simulink model "RefModel_Navfilter"  (R2020b)
settings: Solver=ode1  StartTime=0.0  StopTime=inf  FixedStep=Ts_Navi.Ts_Base  RelTol=1e-3
values from neighbouring files (symbols this model uses):
  NAVI_PARAM_V10 = INIT_Navi_V10(NaviSimParam.Ts_Base)    [SetAlgoParam_Navi.m]
  NAVI_PARAM_V1000 = INIT_Navi_V1000(NaviSimParam.Ts_Base)    [SetAlgoParam_Navi.m]
undefined symbols (not defined in the file or in its folder): ENUM_SensorHealthStatus, NAVI_PARAM_BASE
libraries: aerolibobsolete x1
(part 2 of 2)

== stateflow chart RefModel_Navfilter/Filter_Stateflow ==
  state NaviPlatform
    en:
    initOutputData();
    initMember();
    en,du:
    % 获取输入数据
    getTaskData();
    getSensorData();
    getIntegrityData();
    % 公共状态更新
    updateMember();
    upDataOutputData();
    state LogData [parallel]
      en:
      settings: executionOrder=1
      state Work
        en,du:
        du_func_commonInfo;
        du_func_updateLog;
      (default) -> NaviPlatform.LogData.Work
    state Normal [parallel]
      en,du:
      settings: executionOrder=3
      state InitialWait0
        ex:
        mThis_RTInfo = ENUM_RTInfo_Navi.InitialWait_1_Complete; % 更新RT信息
        updateLogDataBuffer(ENUM_NaviLogBlockName.NAVILOG_Init,mThis_RTInfo,'write',double([mSensor_ublox1_pdop, mSensor_ublox1_numSv, mSensor_ublox1_pacc])); % 更新log缓存
      state InitialWait1
        ex:
        mThis_RTInfo = ENUM_RTInfo_Navi.InitialWait_2_Complete; % 更新RT信息
        updateLogDataBuffer(ENUM_NaviLogBlockName.NAVILOG_Init,mThis_RTInfo,'write',double([mSensor_ublox1_pdop, mSensor_ublox1_numSv, mSensor_ublox1_pacc])); % 更新log缓存
      state InitialAlignment
        en:
        du:
        % 执行初始化，完成滤波器初始状态的确定
        NaviFilterOut.Status.initialAlignmentComplete = coarseAlignment();
        NaviFilterOut.magDec_deg = magDec_deg;
        NaviFilterOut.Status.initNotComplete = 1;
        ex:
        NaviFilterOut.Status.initNotComplete = 0;
        mThis_RTInfo = ENUM_RTInfo_Navi.InitialWait_2_Complete; % 更新RT信息
        updateLogDataBuffer(ENUM_NaviLogBlockName.NAVILOG_Init,mThis_RTInfo,'write',[NaviFilterOut.InitValue.lla0(1:2),NaviFilterOut.InitValue.eulerd0]); % 更新log缓存
      state RunKalmanFilter
        en:
        du:
        du_func_KalmanFilter(NAVIParam.modeKF1); % marg mvo
      (default) -> InitialWait0
      InitialWait0 -> InitialWait1 : [isUbloxGoodForAWhile()]
      InitialWait1 -> InitialAlignment : [after(10,sec) && isUbloxGood()]
      InitialAlignment -> RunKalmanFilter : [isInitComplete()]
    state Radar [parallel]
      % 用于降落阶段雷达高度融合
      settings: executionOrder=2
      state StandBy
        en:
        resetRadarFuser = true;
      state Work
        en:
        height0Ublox1 = double(IN_Sensor.ublox1.height) - double(IN_Sensor.radar1.Range);
        height0Um482 = double(IN_Sensor.um482.height) - double(IN_Sensor.radar1.Range);
        height0Baro1 = double(IN_Sensor.baro1.alt_baro) - double(IN_Sensor.radar1.Range);
        du:
        du_func;
      (default) -> StandBy
      StandBy -> NaviPlatform.Radar.Work : [isRadarReady && after(0.1,sec)]
      NaviPlatform.Radar.Work -> StandBy : [~isRadarReady && after(2,sec)]
  data: blockName function_input; message function_input; operation function_input; varargin function_input; accel function_output; gyro function_output; imuUpdateFlag function_output; flag function_output; flag function_output; vel function_input; flag function_output; flag function_output; heading function_input; heading_ecompass function_input; flag function_output; isSuccess function_output; mode function_input; flag function_output; x_out function_output; Vd function_input; height function_input; Ts_in function_input; P_out function_output; dz_out function_output; Pz_out function_output; reset function_input; reject_threshold function_input; Q function_input; R function_input; mode function_input; mag function_output; magUpdateFlag function_output; isBagMag function_output; tas function_output; airspeedUpdateFlag function_output; alt function_output; baroUpdateFlag function_output; range function_output; radarUpdateFlag function_output; out function_output; Ts input; clock_sec input; magDec_deg input; IN_Sensor input Bus: BUS_SENSOR; IN_SignalIntegrity input Bus: BUS_NAVI_SensorSignalIntegrity; IN_Task input size=1; mThis_bestpos local Enum: ENUM_BESTPOS; isBadAttitude local; resetRadarFuser local; RadarFilterOut output Bus: BUS_NAVI_RadarFilter size=1; MVOParam data_store_memory; height0Baro1 local; height0Ublox1 local; height0Um482 local; NaviFilterOut output Bus: BUS_NAVI_FilterOut size=1; MARGParam data_store_memory; NAVIParam data_store_memory; isDebugInfoToShow data_store_memory; mThis_RTInfo local Enum: ENUM_RTInfo_Navi =ENUM_RTInfo_Navi(0); logDataBuffer output Bus: BUS_NAVI_SingleLog size=32; logDataOut output Bus: BUS_NAVI_SingleLog size=1; mSensor_radar1_range local; mSensor_baro1_alt local; mSensor_airspeed1_ias local; mSensor_um482_bestpos local; mSensor_IMU1_acc local; mSensor_IMU1_gyro local; mSensor_IMU2_acc local; mSensor_IMU3_acc local; mSensor_IMU2_gyro local; mSensor_IMU3_gyro local; mSensor_mag1_mag local; mSensor_mag2_mag local; mSensor_ublox1_lla local; mSensor_ublox1_ll local; mSensor_ublox1_lat local; mSensor_ublox1_lon local; mSensor_ublox1_gpsvel local; mSensor_ublox1_vd local; mSensor_ublox1_alt local; mSensor_ublox1_pdop local; mSensor_ublox1_pacc local; mSensor_ublox1_sacc local; mSensor_ublox1_numSv local; mSensor_ublox1_groundSpeed local; mSensor_airspeed2_ias local; mSensor_airspeed3_ias local; mSensor_um482_lat local; mSensor_um482_lon local; mSensor_um482_alt local; mSensor_um482_lla local; mSensor_um482_ll local; mSensor_um482_gpsvel local; mSensor_um482_groundSpeed local; mSensor_um482_vd local; mSensor_um482_pdop local; mSensor_um482_pacc local; mSensor_um482_numSv local; mIntegrity_select_IMU local; mIntegrity_statusSystemHealth local; mIntegrity_status_radar1 local; mIntegrity_status_ublox1 local; mIntegrity_status_um482 local; mIntegrity_status_airspeed1 local; mIntegrity_select_mag local; mIntegrity_select_airspeed local; mIntegrity_select_baro local; mIntegrity_select_radar local; mIntegrity_select_camera local; mIntegrity_status_mag1 local; mIntegrity_status_mag2 local; mIntegrity_status_IMU1 local; mIntegrity_status_IMU2 local; mIntegrity_status_IMU3 local; mIntegrity_status_airspeed2 local; mIntegrity_update_IMU1 local; mIntegrity_update_IMU2 local; mIntegrity_update_IMU3 local; mIntegrity_update_mag1 local; mIntegrity_update_mag2 local; mIntegrity_update_ublox1 local; mIntegrity_update_um482 local; mIntegrity_update_baro1 local; data local; mIntegrity_update_radar1 local; mIntegrity_update_radar2 local; mIntegrity_update_radar3 local; mIntegrity_update_airspeed1 local; mIntegrity_update_airspeed2 local; mIntegrity_update_airspeed3 local; mIntegrity_status_baro1 local; mTask_taskMode local
  function initOutputData:
    | function initOutputData
    | % 输出结构体进行赋值，避免报"调用前没有赋值"的错误，每个结构体赋值1个成员即可
    | NaviFilterOut.Status.initNotComplete = int8(1);
    | logDataOut(1).time_sec = 0;
    | logDataBuffer(1).time_sec = 0;
  function initMember:
    | function initMember()
    | % 初始化成员变量
  function upDataOutputData:
    | function upDataOutputData
    | % 
    | NaviFilterOut.magDec_deg = magDec_deg;
    | NaviFilterOut.hitGroundByAccZ = isHitGround(mSensor_IMU1_acc,Ts);
    | 
    | %% 子函数
    | function flag = isHitGround(acc, Ts)
    | persistent duration
    | if isempty(duration)
    |     duration = 0;
    | end
    | hitSuccess = acc(3)>14;
    | flag = true;
    | if not( hitSuccess ) 
    |     duration = duration + Ts;
    |     if duration > 0.5 % 没有出现大az一段时间后,false
    |         flag = false;
    |     end 
    | else % 出现大az，true
    |     flag = true;
    |     duration = 0;
    | end
  function updateMember:
    | function updateMember()
    | %% 每时刻均需计算的成员在此计算，大部分成员在子级模块中更新
    | %% 更新成员变量
    | mThis_bestpos = enumBESTPOS();
  function getIntegrityData:
    | function getIntegrityData()
    | % 输入结构体
    | %% 直接量
    | % 通道选择
    | mIntegrity_select_IMU = IN_SignalIntegrity.SensorSelect.IMU;
    | mIntegrity_select_mag = IN_SignalIntegrity.SensorSelect.Mag;
    | mIntegrity_select_airspeed = IN_SignalIntegrity.SensorSelect.Airspeed;
    | mIntegrity_select_baro = IN_SignalIntegrity.SensorSelect.Baro;
    | mIntegrity_select_radar = IN_SignalIntegrity.SensorSelect.Radar;
    | mIntegrity_select_camera = IN_SignalIntegrity.SensorSelect.Camera;
    | % 健康状态
    | mIntegrity_statusSystemHealth = IN_SignalIntegrity.SystemHealthStatus;
    | 
    | mIntegrity_status_IMU1 = IN_SignalIntegrity.SensorStatus.IMU1;
    | mIntegrity_status_IMU2 = IN_SignalIntegrity.SensorStatus.IMU2;
    | mIntegrity_status_IMU3 = IN_SignalIntegrity.SensorStatus.IMU3;
    | mIntegrity_status_mag1 = IN_SignalIntegrity.SensorStatus.mag1;
    | mIntegrity_status_mag2 = IN_SignalIntegrity.SensorStatus.mag2;
    | mIntegrity_status_radar1 = IN_SignalIntegrity.SensorStatus.radar1;
    | mIntegrity_status_baro1 = IN_SignalIntegrity.SensorStatus.baro1;
    | mIntegrity_status_ublox1 = IN_SignalIntegrity.SensorStatus.ublox1;
    | mIntegrity_status_um482 = IN_SignalIntegrity.SensorStatus.um482;
    | mIntegrity_status_airspeed1 = IN_SignalIntegrity.SensorStatus.airspeed1;
    | % 更新标志
    | mIntegrity_update_IMU1 = IN_SignalIntegrity.SensorUpdateFlag.IMU1;
    | mIntegrity_update_IMU2 = IN_SignalIntegrity.SensorUpdateFlag.IMU2;
    | mIntegrity_update_IMU3 = IN_SignalIntegrity.SensorUpdateFlag.IMU3;
    | mIntegrity_update_mag1 = IN_SignalIntegrity.SensorUpdateFlag.mag1;
    | mIntegrity_update_mag2 = IN_SignalIntegrity.SensorUpdateFlag.mag2;
    | mIntegrity_update_ublox1 = IN_SignalIntegrity.SensorUpdateFlag.ublox1;
    | mIntegrity_update_um482 = IN_SignalIntegrity.SensorUpdateFlag.um482;
    | mIntegrity_update_baro1 = IN_SignalIntegrity.SensorUpdateFlag.baro1;
    | mIntegrity_update_radar1 = IN_SignalIntegrity.SensorUpdateFlag.radar1;
    | mIntegrity_update_radar2 = IN_SignalIntegrity.SensorUpdateFlag.radar2;
    | mIntegrity_update_radar3 = IN_SignalIntegrity.SensorUpdateFlag.radar3;
    | mIntegrity_update_airspeed1 = IN_SignalIntegrity.SensorUpdateFlag.airspeed1;
    | mIntegrity_update_airspeed2 = IN_SignalIntegrity.SensorUpdateFlag.airspeed2;
    | mIntegrity_update_airspeed3 = IN_SignalIntegrity.SensorUpdateFlag.airspeed3;
    | %% 间接量
  function getSensorData:
    | function getSensorData
    | %% 输入结构体
    | %% 直接量
    | % IMU
    | mSensor_IMU1_az = IN_Sensor.IMU1.accel_z;
    | mSensor_IMU1_acc = double([IN_Sensor.IMU1.accel_x,IN_Sensor.IMU1.accel_y,IN_Sensor.IMU1.accel_z]);
    | mSensor_IMU2_acc = double([IN_Sensor.IMU2.accel_x,IN_Sensor.IMU2.accel_y,IN_Sensor.IMU2.accel_z]);
    | mSensor_IMU3_acc = double([IN_Sensor.IMU3.accel_x,IN_Sensor.IMU3.accel_y,IN_Sensor.IMU3.accel_z]);
    | 
    | mSensor_IMU1_gyro = double([IN_Sensor.IMU1.gyro_x,IN_Sensor.IMU1.gyro_y,IN_Sensor.IMU1.gyro_z]);
    | mSensor_IMU2_gyro = double([IN_Sensor.IMU2.gyro_x,IN_Sensor.IMU2.gyro_y,IN_Sensor.IMU2.gyro_z]);
    | mSensor_IMU3_gyro = double([IN_Sensor.IMU3.gyro_x,IN_Sensor.IMU3.gyro_y,IN_Sensor.IMU3.gyro_z]);
    | % 磁力计
    | mSensor_mag1_mag = double([IN_Sensor.mag1.mag_x, IN_Sensor.mag1.mag_y, IN_Sensor.mag1.mag_z]);
    | mSensor_mag2_mag = double([IN_Sensor.mag2.mag_x, IN_Sensor.mag2.mag_y, IN_Sensor.mag2.mag_z]);
    | % 雷达高度计
    | mSensor_radar1_range = double(IN_Sensor.radar1.Range);
    | % 气压高度计
    | mSensor_baro1_alt = double(IN_Sensor.baro1.alt_baro);
    | % 空速计
    | mSensor_airspeed1_ias = double(IN_Sensor.airspeed1.airspeed_indicate);
    | mSensor_airspeed2_ias = double(IN_Sensor.airspeed2.airspeed_indicate);
    | mSensor_airspeed3_ias = double(IN_Sensor.airspeed3.airspeed_indicate);
    | % um482
    | mSensor_um482_bestpos = IN_Sensor.um482.BESTPOS;
    | % ublox
    | gpsStruct = IN_Sensor.ublox1;
    | mSensor_ublox1_lat = double(gpsStruct.Lat);
    | mSensor_ublox1_lon = double(gpsStruct.Lon);
    | mSensor_ublox1_alt = double(gpsStruct.height);
    | mSensor_ublox1_lla = [mSensor_ublox1_lat, mSensor_ublox1_lon, mSensor_ublox1_alt];
    | mSensor_ublox1_ll = [mSensor_ublox1_lat, mSensor_ublox1_lon];
    | mSensor_ublox1_gpsvel = double([gpsStruct.velN, gpsStruct.velE, gpsStruct.velD]);
    | mSensor_ublox1_groundSpeed = norm(mSensor_ublox1_gpsvel);
    | mSensor_ublox1_vd = double(gpsStruct.velD);
    | mSensor_ublox1_pdop = gpsStruct.pDop;
    | mSensor_ublox1_pacc = double([gpsStruct.hAcc,gpsStruct.hAcc,gpsStruct.vAcc]);
    | mSensor_ublox1_sacc = double(gpsStruct.sAcc);
    | mSensor_ublox1_numSv = gpsStruct.numSv;
    | % um482
    | gpsStruct = IN_Sensor.um482;
    | mSensor_um482_lat = double(gpsStruct.Lat);
    | mSensor_um482_lon = double(gpsStruct.Lon);
    | mSensor_um482_alt = double(gpsStruct.height);
    | mSensor_um482_lla = [mSensor_um482_lat, mSensor_um482_lon, mSensor_um482_alt];
    | mSensor_um482_ll = [mSensor_um482_lat, mSensor_um482_lon];
    | mSensor_um482_gpsvel = double([gpsStruct.velN, gpsStruct.velE, gpsStruct.velD]);
    | mSensor_um482_groundSpeed = norm(mSensor_um482_gpsvel);
    | mSensor_um482_vd = double(gpsStruct.velD);
    | mSensor_um482_pdop = double(gpsStruct.pDop);
    | mSensor_um482_pacc = double([gpsStruct.delta_lat,gpsStruct.delta_lon,gpsStruct.delta_height]);
    | mSensor_um482_numSv = gpsStruct.numSv;
    | mSensor_um482_bestpos = gpsStruct.BESTPOS;
    | %% 间接量
  function getTaskData:
    | function getTaskData()
    | %% 输入结构体
    | %% 直接量
    | mTask_taskMode = IN_Task.flightTaskMode;
    | %% 间接量
  function updateLogDataBuffer(blockName,message,operation,varargin):
    | function updateLogDataBuffer(blockName,message,operation,varargin)
    | persistent pIdx pBufferIdx preTime
    | if isempty(pIdx)
    |     pIdx = 0;
    |     pBufferIdx = 0;
    |     preTime = clock_sec;
    | end
    | %%
    | if nargin == 4
    |     var_input = reshape(varargin{1},5,1);
    | else
    |     var_input = zeros(5,1);
    | end
    | bufferIdx = pBufferIdx;
    | idx = pIdx;
    | thisTime = clock_sec;
    | switch operation
    |     case 'write'
    |         thisTime = clock_sec;
    |         if preTime ~= thisTime
    |             idx = 0; % 同一时间刻度下, 不同信息的先后顺序
    |         end
    |         if bufferIdx < length(logDataBuffer)
    |             bufferIdx = bufferIdx + 1;
    |             idx = idx + 1;
    |             temp = formatLogStruct(blockName,message,var_input);
    |             tempData.time_sec = clock_sec;
    |             tempData.idx = idx;
    |             tempData.blockName = blockName;
    |             tempData.message = message;
    |             tempData.var1 = temp.var1;
    |             logDataBuffer(bufferIdx) = tempData;            
    |         end
    |     case 'read'
    |         for i_out = 1:1 %AlgoParams.logDataOutSize
    |             %             logDataOut(i_out) = resetLogStruct; % 置零
    |             logDataOut(i_out).time_sec = 0;
    |             logDataOut(i_out).idx = 0;
    |             logDataOut(i_out).blockName = ENUM_NaviLogBlockName(0);
    |             logDataOut(i_out).message = ENUM_RTInfo_Navi(0);
    |             logDataOut(i_out).var1 = zeros(5,1);
    |             if bufferIdx > 0
    |                 % 读取当前数据
    |                 logDataOut(i_out) = logDataBuffer(bufferIdx);
    |                 %                 logDataBuffer(bufferIdx) = resetLogStruct;
    | %                 fprintf('read time \t idx \t block \t message \t var1\n%.3f \t %.0f \t %d \t %d \t %.3f\n',...
    | %                     logDataBuffer(bufferIdx).time_sec,...
    | %                     logDataBuffer(bufferIdx).idx,...
    | %                     int16(logDataBuffer(bufferIdx).blockName),...
    | %                     int16(logDataBuffer(bufferIdx).message),...
    | %                     logDataBuffer(bufferIdx).var1(1));
    |                 % 将当前位置数据置零
    |                 logDataBuffer(bufferIdx).time_sec = 0;
    |                 logDataBuffer(bufferIdx).idx = 0;
    |                 logDataBuffer(bufferIdx).blockName = ENUM_NaviLogBlockName(0);
    |                 logDataBuffer(bufferIdx).message = ENUM_RTInfo_Navi(0);
    |                 logDataBuffer(bufferIdx).var1 = zeros(5,1);
    |                 bufferIdx = bufferIdx - 1;
    |             end
    |         end
    | end
    | % fprintf("logbuffer  %d / %d\n", int16(bufferIdx), int16(length(logDataBuffer)));
    | preTime = thisTime;
    | pBufferIdx = bufferIdx;
    | pIdx = idx;
    | %% 子函数
    | function log = formatLogStruct(blockName,message,var_input)
    | log.message = message;
    | log.var1 = zeros(5,1);
    | % switch blockName
    | %     case ENUM_TaskLogBlockName.TASKLOG_FlightMode
    | %         log.var1(1) = ComFlightOut.curLLA(1);
    | %         log.var1(2) = ComFlightOut.curLLA(2);
    | %         log.var1(3) = ComFlightOut.curLLA(3);
    | %         log.var1(4) = norm(ComFlightOut.curAirSpeed);
    | %         log.var1(5) = PathModeOut.uavMode;
    | % end
    | % log.var1(5) = double(IN_Mav.mavlink_msg_mission_current(1).remaining)/100;
    | if sum(var_input) ~= 0
    |     log.var1 = var_input; % 输入的优先级高
    | end
  function [accel,gyro,imuUpdateFlag] = getScreeningIMU:
    | function [accel,gyro,imuUpdateFlag] = getScreeningIMU()
    | if mIntegrity_select_IMU == 1
    |     imuUpdateFlag = mIntegrity_update_IMU1;
    |     accel = mSensor_IMU1_acc;
    |     gyro = mSensor_IMU1_gyro;
    | elseif mIntegrity_select_IMU == 2
    |     imuUpdateFlag = mIntegrity_update_IMU2;
    |     accel = mSensor_IMU2_acc;
    |     gyro = mSensor_IMU2_gyro;
    | elseif mIntegrity_select_IMU == 3
    |     imuUpdateFlag = mIntegrity_update_IMU3;
    |     accel = mSensor_IMU3_acc;
    |     gyro = mSensor_IMU3_gyro;
    | elseif mIntegrity_select_IMU == 0
    |     imuUpdateFlag = mIntegrity_update_IMU1 || mIntegrity_update_IMU2 || mIntegrity_update_IMU3;
    |     accel = (mSensor_IMU1_acc+mSensor_IMU2_acc+mSensor_IMU3_acc)/3;
    |     gyro = (mSensor_IMU1_gyro+mSensor_IMU2_gyro+mSensor_IMU3_gyro)/3;
    | else
    |     imuUpdateFlag = true;
    |     accel = [0,0,0];
    |     gyro = [0,0,0];
    |     error('IMU config error')
    | end
  function du_func_commonInfo:
    | function du_func_commonInfo
  function du_func_updateLog:
    | function du_func_updateLog
    | updateLogDataBuffer(ENUM_NaviLogBlockName.NAVILOG_None,ENUM_RTInfo_Navi(0),'read')
  function flag = isUbloxGood:
    | function flag = isUbloxGood
    | flag = false;
    | if mSensor_ublox1_pdop <= 3 && mSensor_ublox1_pdop ~= 0 && mSensor_ublox1_numSv >= 10
    |     flag = true;
    | end
  function flag = isMoving(vel):
    | function flag = isMoving(vel)
    | % 运动判断
    | persistent preSpeed
    | speed = norm(vel);
    | if isempty(preSpeed)
    |     preSpeed = speed;
    | end
    | k = 0.9;
    | preSpeed = k*preSpeed + (1-k)*speed;
    | flag = false;
    | if preSpeed > 0.5
    |     flag = true; 
    | end
  function flag = isUbloxGoodForAWhile:
    | function flag = isUbloxGoodForAWhile
    | persistent duration
    | if isempty(duration)
    |     duration = 0;
    | end
    | 
    | flag = false;
    | 
    | if isUbloxGood
    |     duration = duration + Ts;
    |     if duration > 5 % sec
    | %         fprintf('ublox pDOP<3 for 5sec.\n');
    |         flag = true;
    |     end
    | else
    |     duration = 0;
    | end
  function flag = isHeadingRotate(heading,heading_ecompass):
    | function flag = isHeadingRotate(heading,heading_ecompass)
    | % 航向估计异常自旋判定
    | persistent dHeadingSet preHeadingVal duration du_fprintf meanDotHeading headingErr
    | if isempty(dHeadingSet)
    |     dHeadingSet = nan(8,1);
    |     preHeadingVal = heading;
    |     duration = 0;
    |     du_fprintf = 0;
    |     meanDotHeading = 0;
    |     headingErr = 0;
    | end
    | duration = duration + Ts;
    | du_fprintf = du_fprintf + Ts;
    | %% 计算航向角速度
    | dt = 1.5; % sec
    | if duration >= dt
    |     dHeading = angdiff(heading,preHeadingVal)/dt;
    |     preHeadingVal = heading;
    |     dHeadingSet(1:end-1) = dHeadingSet(2:end);
    |     dHeadingSet(end) = dHeading;
    |     duration = 0;
    | end
    | %% 判断是否异常自旋
    | flag = false;
    | if all(~isnan(dHeadingSet))
    |     meanDotHeading = mean(dHeadingSet);
    |     if abs(meanDotHeading) > 0.5*pi/180
    |         flag = true;
    |     end
    | end
    | %% EKF滤波heading 和 ecompass heading的比较
    | % if TaskMode == ENUM_FlightTaskMode.GroundStandByMode
    |     headingErr = abs(angdiff(heading,heading_ecompass));
    |     if headingErr > 20*pi/180
    |         flag = true;
    |     end
    | % end
    | %%
    | if du_fprintf > 5
    |     du_fprintf = 0;
    |     fprintf('meanDotHeading: %.2f deg/s\t\t',meanDotHeading*57.3);
    |     fprintf('headingErr: %.1f deg\n',headingErr*57.3);
    | %     if clock_sec > 290
    | %         sl = 1;
    | %     end
    | end
  function flag = isInitComplete:
    | function flag = isInitComplete()
    | flag = NaviFilterOut.Status.initialAlignmentComplete;
  function isSuccess = coarseAlignment:
    | function isSuccess = coarseAlignment()
    | persistent eulerd_buffer baro1_alt_buffer radar1_range_buffer quat_buffer curEulerd
    | persistent ublox1_lla_buffer ublox1_gpsvel_buffer um482_lla_buffer um482_gpsvel_buffer
    | persistent IMU_acc_buffer IMU_gyro_buffer
    | persistent mag_buffer
    | persistent internalTime
    | persistent isBadAttitude0 preMagNum
    | persistent pInitNum
    | % 数据初始化
    | bufferSize = 50;
    | bufferSizeGPS = 10;
    | flag = 9999;
    | thisMagNum = mIntegrity_select_mag;
    | if isempty(preMagNum)
    |     preMagNum = thisMagNum;
    | end
    | if isempty(pInitNum)
    |     pInitNum = 0;
    | end
    | if thisMagNum == preMagNum
    |     isTheSameMag = true;
    | else
    |     isTheSameMag = false;
    | end
    | isRestartInit = mSensor_ublox1_pdop > 3 || ...
    |      mIntegrity_select_mag < 0;
    | %      || ~isTheSameMag;
    | if isempty(IMU_acc_buffer) || isRestartInit
    |     pInitNum = pInitNum + 1;
    |     eulerd_buffer = flag*ones(bufferSize,3);
    |     quat_buffer = flag*ones(bufferSize,4);
    |     
    |     baro1_alt_buffer = flag*ones(1,bufferSize);
    |     radar1_range_buffer = flag*ones(1,bufferSize);
    |     
    |     ublox1_lla_buffer = flag*ones(bufferSizeGPS,3);
    |     ublox1_gpsvel_buffer = flag*ones(bufferSizeGPS,3);
    |     um482_lla_buffer = flag*ones(bufferSizeGPS,3);
    |     um482_gpsvel_buffer = flag*ones(bufferSizeGPS,3);
    |     
    |     IMU_acc_buffer = flag*ones(bufferSize,3);
    |     IMU_gyro_buffer = flag*ones(bufferSize,3);
    |     
    |     mag_buffer = flag*ones(bufferSize,3);
    |     internalTime = 0;
    |     nMagDegrade = 0;
    |     isBadAttitude0 = 0;
    |     preMagNum = thisMagNum;
    |     curEulerd = flag*ones(bufferSize,3);
    |     fprintf('Init Number: %.0f\n',pInitNum);
    | end
    | NaviFilterOut.Status.initNum = pInitNum;
    | preMagNum = thisMagNum;
    | internalTime = internalTime + Ts;
    | 
    | std_acc = zeros(1,3);
    | std_gyro = zeros(1,3);
    | std_mag = zeros(1,3);
    | std_lla = zeros(1,3);
    | std_gpsvel = zeros(1,3);
    | std_alt = zeros(1,1);
    | std_range = zeros(1,1);
    | %% 传感器数据池更新
    | if mIntegrity_update_IMU1
    |     IMU_acc_buffer(1:bufferSize-1,:) = IMU_acc_buffer(2:bufferSize,:);
    |     IMU_acc_buffer(bufferSize,:) = mSensor_IMU1_acc;
    |     IMU_gyro_buffer(1:bufferSize-1,:) = IMU_gyro_buffer(2:bufferSize,:);
    |     IMU_gyro_buffer(bufferSize,:) = mSensor_IMU1_gyro;
    | end
    | 
    | % 更新IMU
    | IMU_acc_buffer(1:bufferSize-1,:) = IMU_acc_buffer(2:bufferSize,:);
    | IMU_gyro_buffer(1:bufferSize-1,:) = IMU_gyro_buffer(2:bufferSize,:);
    | [accelTemp,gyroTemp,imuUpdateFlag] = getScreeningIMU();
    | if imuUpdateFlag
    |     IMU_acc_buffer(bufferSize,:) = accelTemp;
    |     IMU_gyro_buffer(bufferSize,:) = gyroTemp;
    | end
    | % 更新GPS
    | if mIntegrity_update_ublox1
    |     if ~isequal(mSensor_ublox1_lla,[0,0,0])
    |         ublox1_lla_buffer(1:bufferSizeGPS-1,:) = ublox1_lla_buffer(2:bufferSizeGPS,:);
    |         ublox1_lla_buffer(bufferSizeGPS,:) = mSensor_ublox1_lla;
    |         ublox1_gpsvel_buffer(1:bufferSizeGPS-1,:) = ublox1_gpsvel_buffer(2:bufferSizeGPS,:);
    |         ublox1_gpsvel_buffer(bufferSizeGPS,:) = mSensor_ublox1_gpsvel;
    |     end
    | end
    | if mIntegrity_update_um482
    |     if ~isequal(mSensor_um482_lla,[0,0,0])
    |         um482_lla_buffer(1:bufferSizeGPS-1,:) = um482_lla_buffer(2:bufferSizeGPS,:);
    |         um482_lla_buffer(bufferSizeGPS,:) = mSensor_um482_lla;
    |         um482_gpsvel_buffer(1:bufferSizeGPS-1,:) = um482_gpsvel_buffer(2:bufferSizeGPS,:);
    |         um482_gpsvel_buffer(bufferSizeGPS,:) = mSensor_um482_gpsvel;
    |     end
    | end
    | if mIntegrity_update_baro1
    |     baro1_alt_buffer(1:bufferSize-1) = baro1_alt_buffer(2:bufferSize);
    |     baro1_alt_buffer(bufferSize) = mSensor_baro1_alt;
    | end
    | if mIntegrity_update_radar1
    |     radar1_range_buffer(1:bufferSize-1) = radar1_range_buffer(2:bufferSize);
    |     radar1_range_buffer(bufferSize) = mSensor_radar1_range;
    | end
    | % 更新姿态
    | mag_buffer(1:bufferSize-1,:) = mag_buffer(2:bufferSize,:);
    | quat_buffer(1:bufferSize-1,:) = quat_buffer(2:bufferSize,:);
    | eulerd_buffer(1:bufferSize-1,:) = eulerd_buffer(2:bufferSize,:);
    | [curMag,magUpdateFlag,isBadAttitude0] = getScreeningMag();
    | if magUpdateFlag
    |     mag_buffer(bufferSize,:) = curMag;
    |     quat_buffer(bufferSize,:) = compact(ecompass(IMU_acc_buffer(bufferSize,:),mag_buffer(bufferSize,:)));
    |     curEulerd = eulerd(quat_buffer(bufferSize,:));
    |     eulerd_buffer(bufferSize,:) = curEulerd;
    | end
    | %% 初始化条件判定
    | tmax = 300; % 最大初始化时间
    | posStable_threshold = 3;
    | attitudeStable_threshold = 2; % deg
    | llaStable_threshold = [1e-5*posStable_threshold,1e-5*posStable_threshold,10]; % deg deg m
    | gyroStable_threshold = 2*pi/180; % rad
    | gyroMax_threshold = 3*pi/180; % rad
    | accStable_threshold = 0.5;
    | initCondition.attitudeStable = std(eulerd_buffer(:,2)) < attitudeStable_threshold && ...
    |     std(eulerd_buffer(:,3)) < attitudeStable_threshold;
    | % std(eulerd_buffer(:,1)) < attitudeStable_threshold 航向会有180度跳变问题
    | initCondition.LLAStable = std(ublox1_lla_buffer(:,1)) < llaStable_threshold(1) && ...
    |     std(ublox1_lla_buffer(:,2)) < llaStable_threshold(2) && ...
    |     std(ublox1_lla_buffer(:,3)) < llaStable_threshold(3);
    | initCondition.gyroStable = std(IMU_gyro_buffer(:,1)) < gyroStable_threshold  && ...
    |     std(IMU_gyro_buffer(:,2)) < gyroStable_threshold  && ...
    |     std(IMU_gyro_buffer(:,3)) < gyroStable_threshold  && ...
    |     mean(IMU_gyro_buffer(:,1)) < gyroMax_threshold && ...
    |     mean(IMU_gyro_buffer(:,2)) < gyroMax_threshold && ...
    |     mean(IMU_gyro_buffer(:,3)) < gyroMax_threshold;
    | initCondition.accStable = std(IMU_acc_buffer(:,1)) < accStable_threshold  && ...
    |     std(IMU_acc_buffer(:,2)) < accStable_threshold  && ...
    |     std(IMU_acc_buffer(:,3)) < accStable_threshold ;
    | initCondition.attitudeNorminal = abs(mean(eulerd_buffer(:,1))) < 400 && ...
    |     abs(max(eulerd_buffer(:,2))) < 45 && ...
    |     abs(max(eulerd_buffer(:,3))) < 45 && ...
    |     abs(curEulerd(2)) < 45 && ...
    |     abs(curEulerd(3)) < 45;
    | initCondition.LLANorminal = abs(mean(ublox1_lla_buffer(:,1))) < 90 && ...
    |     abs(mean(ublox1_lla_buffer(:,2))) < 180 && ...
    |     abs(mean(ublox1_lla_buffer(:,3))) < 20e3;
    | if (internalTime > tmax/2) && abs(mean(mag_buffer(:,1))-flag)<1e-5 % 初始化时长大于tmax/2，且磁力计未更新
    |     eulerd_buffer = zeros(bufferSize,3);
    |     initCondition.attitudeStable = true;
    |     initCondition.attitudeNorminal = true;
    |     isBadAttitude0 = 1;
    | end
    | initCondition.altNorminal = std(baro1_alt_buffer) < 5 && ...
    |     abs(mean(baro1_alt_buffer)) < flag/2;
    | initCondition.UavStable = false;
    | initCondition.AllSensorNorminal = false;
    | initCondition.AllSensorNorminal = initCondition.attitudeNorminal && ...
    |     initCondition.LLANorminal && ...
    |     initCondition.altNorminal;
    | initCondition.UavStable = initCondition.attitudeStable &&... % 姿态稳定要求
    |     initCondition.LLAStable &&... % 位置稳定要求
    |     initCondition.gyroStable &&...  % 角速度稳定要求
    |     initCondition.accStable &&... % 加速度稳定要求
    |     initCondition.AllSensorNorminal;
    | isBadAttitude = isBadAttitude0;
    | isSuccess = false; % 初始化成功标志
    | if initCondition.UavStable || ...% 标准解锁
    |         (internalTime > tmax && initCondition.AllSensorNorminal)% 特殊解锁1
    |     fprintf('%.3f sec: NavFilter Init Complete\n',clock_sec);
    |     isSuccess = true;
    |     % 均值
    |     acc_bias0 = mean(IMU_acc_buffer,1);
    |     dw0 = mean(IMU_gyro_buffer,1);
    |     alt0 = mean(ublox1_lla_buffer(:,3));
    |     pos0_ublox1 = mean(ublox1_lla_buffer,1); % LLA (deg deg m)
    |     gpsvel0_ublox1 = mean(ublox1_gpsvel_buffer,1);
    |     range0 = mean(radar1_range_buffer);
    |     eulerd0 = mean(eulerd_buffer,1);
    |     eulerd0(1) = eulerd_buffer(end,1);
    |     % 方差
    |     std_acc = std(IMU_acc_buffer,[],1);
    |     std_gyro = std(IMU_gyro_buffer,[],1);
    |     std_mag = std(mag_buffer,[],1);
    |     temp = std(ublox1_lla_buffer,[],1);
    |     std_lla = [111e3*cos(pi/180*pos0_ublox1(1)),111e3,1].*temp;
    |     std_gpsvel = std(ublox1_gpsvel_buffer,[],1);
    |     std_alt = std(baro1_alt_buffer);
    |     std_range = std(radar1_range_buffer);
    |     % 确定初始
    |     NaviFilterOut.InitValue.acc_bias0 = acc_bias0;
    |     if all(abs(dw0) < 1*pi/180)
    |         NaviFilterOut.InitValue.gyro_bias0 = dw0;
    |     else
    |         NaviFilterOut.InitValue.gyro_bias0 = 0*dw0;
    |     end
    |     NaviFilterOut.InitValue.alt0 = alt0;
    |     % 确定位置初值
    |     gpsMode = selectGPSsource(mThis_bestpos,MARGParam.fuse_enable.um482);
    |     switch gpsMode
    |         case 'ublox'
    |             NaviFilterOut.InitValue.lla0 = pos0_ublox1;
    |             NaviFilterOut.InitValue.gpsvel0 = gpsvel0_ublox1;
    |         case 'um482'
    |             NaviFilterOut.InitValue.lla0 = mSensor_um482_lla;
    |             NaviFilterOut.InitValue.gpsvel0 = mSensor_um482_gpsvel;
    |         otherwise
    |             NaviFilterOut.InitValue.lla0 = pos0_ublox1;
    |             NaviFilterOut.InitValue.gpsvel0 = gpsvel0_ublox1;
    |     end
    |     if norm(gpsvel0_ublox1) < 0.5
    |         NaviFilterOut.InitValue.gpsvel0 = [0,0,0];
    |     end
    |     % 
    |     NaviFilterOut.InitValue.range0 = range0;
    |     % 初始姿态
    |     if ~isBadAttitude == 1
    |         NaviFilterOut.InitValue.eulerd0 = eulerd0+[magDec_deg,0,0];
    |     else
    |         NaviFilterOut.InitValue.eulerd0 = [90,0,0];
    |     end
    |     NaviFilterOut.InitValue.quat0 = compact(quaternion(NaviFilterOut.InitValue.eulerd0,'eulerd','ZYX','frame'));
    |     %
    |     NaviFilterOut.InitValue.magNED0 = rotateframe(conj(quaternion(NaviFilterOut.InitValue.quat0)),mean(mag_buffer,1));
    |     NaviFilterOut.InitValue.refloc = NaviFilterOut.InitValue.lla0;
    | end
    | end
    | %% 子函数 ------------------------------------------
    | function eout = eulerd(quat)
    | % rotate 'ZYX'
    | qa = quat(1);
    | qb = quat(2);
    | qc = quat(3);
    | qd = quat(4);
    | the1 = 1;
    | the2 = 2;
    | 
    | tmp = qb.*qd.*the2 - qa.*qc.*the2;
    | if tmp > the1
    |     tmp = the1;
    | elseif tmp < -the1
    |     tmp = -the1;
    | end
    | % tmp(tmp > the1) = the1;
    | % tmp(tmp < -the1) = -the1;
    | b = -asin(tmp);
    | a = atan2((qa.*qd.*the2 + qb.*qc.*the2),(qa.^2.*the2 - the1 + qb.^2.*the2));
    | c = atan2((qa.*qb.*the2 + qc.*qd.*the2),(qa.^2.*the2 - the1 + qd.^2.*the2));
    | % a :  yaw
    | % b :  pitch
    | % c :  roll
    | eout = [a b c]*180/pi;
    | end
    | %
    | function out = selectGPSsource(postype,um482flag)
    | % postype = ENUM_BESTPOS.POS_SOLUTION_SINGLE;
    | if (postype == ENUM_BESTPOS.POS_SOLUTION_PSRDIFF || ...
    |         postype == ENUM_BESTPOS.POS_SOLUTION_L1_INT || ...
    |         postype == ENUM_BESTPOS.POS_SOLUTION_WIDE_INT || ...
    |         postype == ENUM_BESTPOS.POS_SOLUTION_NARROW_INT || ...
    |         postype == ENUM_BESTPOS.POS_SOLUTION_L1_FLOATE || ...
    |         postype == ENUM_BESTPOS.POS_SOLUTION_NARROW_FLOATE) && um482flag
    |     out = 'um482';
    | else
    |     out = 'ublox';
    | end
    | end
  function FilterMARG22:
    | function FilterMARG22()
    | persistent objMARG lla_pre alt_pre range_pre meanAcc meanGyro timeUpdate_ublox
    | persistent step step_imu step_mag step_ublox step_radar step_baro step_board step_tas
    | persistent dHeight_GPS_sub_Baro
    | persistent ublox1_resReject_num um482_resReject_num mag_resReject_num
    | persistent staticTime
    | persistent magRejectForEver
    | persistent pDTime
    | persistent preTaskMode preTAS
    | persistent pEulerd_ecompass
    | persistent idxFuseBaro
    | %%
    | nState = 22; % 
    | %% 传感器数据构造
    | % IMU更新
    | [accel,gyro,imuUpdateFlag] = getScreeningIMU();
    | % Mag更新
    | [mag,magUpdateFlag,isBagMag] = getScreeningMag();
    | % 气压高度计更新
    | [alt,baroUpdateFlag] = getScreeningBaro();
    | % 雷达高度计更新
    | [range,radarUpdateFlag] = getScreeningRadar();
    | % 真空速更新
    | [tas,airspeedUpdateFlag] = getScreeningTAS();
    | % 滤波更新频率：n表示测量数据变化n次后进行一次相应的滤波更新
    | deciIMU = MARGParam.Decimation.imu;
    | deciMag = MARGParam.Decimation.mag;
    | deciBaro = MARGParam.Decimation.baro;
    | deciRadar = MARGParam.Decimation.radar;
    | deciUblox = MARGParam.Decimation.ublox;
    | deciAirspeed = MARGParam.Decimation.airspeed;
    | baseFs = 1/Ts/double(deciIMU);
    | %% 初始化
    | X0_marg22 = [...
    |     NaviFilterOut.InitValue.quat0,...              % 姿态四元数
    |     [0,0,-NaviFilterOut.InitValue.refloc(3)],... % NED位置 【m】
    |     NaviFilterOut.InitValue.gpsvel0,...           % 速度 【m/s】
    |     NaviFilterOut.InitValue.gyro_bias0*Ts,... % 角增量零偏 【rad】
    |     [0,0,0],...                                    % 速度增量零偏 【m/s】
    |     NaviFilterOut.InitValue.magNED0,...       % NED中当地地磁矢量 【uT】
    |     [0,0,0]...                                     % 磁力计零偏 【uT】
    |     ];
    | if isempty(objMARG)
    |     step = 1;
    |     step_imu = 1;
    |     step_mag = 1;
    |     step_ublox = 1;
    |     step_radar = 1;
    |     step_baro = 1;
    |     step_board = 1;
    |     step_tas = 1;
    |     objMARG = NAV_MARG22;%insfilterMARG
    |     objMARG.IMUSampleRate = baseFs;
    |     objMARG.ReferenceLocation = NaviFilterOut.InitValue.refloc;
    |     objMARG.ReferenceLocation(3) = 0;
    |     if nState == 24
    |         objMARG.State = [X0_marg22,0,0];
    |     else
    |         objMARG.State = [X0_marg22];
    |     end
    |     objMARG.AccelerometerBiasNoise = MARGParam.std_acc_bias.^2;
    |     objMARG.AccelerometerNoise = MARGParam.std_acc.^2;
    |     objMARG.GyroscopeBiasNoise = MARGParam.std_gyro_bias.^2;
    |     objMARG.GyroscopeNoise = MARGParam.std_gyro.^2;
    |     objMARG.MagnetometerBiasNoise = MARGParam.std_mag_bias.^2;
    |     objMARG.GeomagneticVectorNoise = MARGParam.std_magNED.^2;
    |     %     if isBadAttitude
    |     MARGParam.P0_MARG(1:4) = [0.2,0.02,0.02,0.1];
    |     %     end    
    |     if nState == 24
    |         P0_windspeed = [3;3].^2;
    |         objMARG.StateCovariance = diag([MARGParam.P0_MARG;P0_windspeed]);
    |     else
    |         objMARG.StateCovariance = diag([MARGParam.P0_MARG]);
    |     end        
    |     lla_pre = mSensor_ublox1_lla;
    |     alt_pre = alt;
    |     range_pre = range;
    |     meanAcc = [0,0,0];
    |     meanGyro = [0,0,0];
    |     meanMag = [0,0,0];
    |     
    |     tmpUbloxLLA = mSensor_ublox1_lla;
    |     dHeight_GPS_sub_Baro = tmpUbloxLLA(3) - alt;
    |     
    |     ublox1_resReject_num = 0;
    |     um482_resReject_num = 0;
    |     mag_resReject_num = 0;
    |     
    |     staticTime = 0;
    |     magRejectForEver = false;
    |     timeUpdate_ublox = clock_sec;
    |     timeUpdate_um482 = clock_sec;
    |     
    |     pDTime = 0;
    |     
    |     preTaskMode = mTask_taskMode;
    |     isRotor2FixComplete = false;
    |     
    |     preTAS = tas;
    |     pEulerd_ecompass = [0 0 0];
    |     
    |     idxFuseBaro = 0; % baro融合次数
    | end
    | %% 若在地面模式下，发生磁力计切换，则重置电磁相关状态
    | thisMagNum = mIntegrity_select_mag;
    | if isReInitMagState(thisMagNum,mTask_taskMode,clock_sec)
    | %     quat0 = filter_marg.State(1:4)';
    |     quat0 = compact(ecompass(accel,mag));
    |     magNED0 = rotateframe(conj(quaternion(quat0)),mag);
    |     idx_gyroBias = 11:13;
    |     idx_magNED = 17:19;
    |     idx_magBias = 20:22;
    |     objMARG.State(idx_gyroBias) = X0_marg22(idx_gyroBias);
    |     objMARG.State(idx_magNED) = magNED0;
    |     objMARG.State(idx_magBias) = 0*objMARG.State(idx_magBias);
    |     MARGParam.P0_MARG(1:4) = [1,0.2,0.2,1];
    |     if nState == 24
    |         objMARG.StateCovariance = diag([MARGParam.P0_MARG;P0_windspeed]);
    |     else
    |         objMARG.StateCovariance = diag([MARGParam.P0_MARG]);
    |     end        
    | end
    | %% 测量协方差
    | Rmag = diag(MARGParam.std_mag.^2);
    | Rpos = diag(MARGParam.std_lla.^2);
    | Rvel = diag(MARGParam.std_gpsvel.^2);
    | Rpos_um482 = diag(MARGParam.std_lla_um482.^2);
    | Rvel_um482 = diag(MARGParam.std_gpsvel_um482.^2);
    | Ralt = MARGParam.std_alt^2;
    | Rrange = MARGParam.std_range^2;
    | Rtas = MARGParam.std_TAS.^2;
    | % GPS 测量精度
    | [Rpos, Rvel] = getUbloxR();
    | [Rpos_um482, Rvel_um482] = getUm482R(Rpos_um482, Rvel_um482);
    | %% 测量值拒绝 （注意：判断上限值应该 包容最大运动能力，下限值应该小于噪声影响）
    | maxSpeed = 30;%30*dt_base;
    | % GPS位置跳变拒绝——判断是否异常跳变
    | posJumpThreshold = maxSpeed; % m
    | m2deg = 1e-5; % 1m vs 1e-5deg
    | measureReject.ublox1_lla_notJump = ...
    |     abs(norm(lla_pre(1)-mSensor_ublox1_lat)) < posJumpThreshold*m2deg || ...
    |     abs(norm(lla_pre(2)-mSensor_ublox1_lon)) < posJumpThreshold*m2deg || ...
    |     abs(norm(lla_pre(3)-mSensor_ublox1_alt)) < posJumpThreshold;
    | % 气压高度位置跳变拒绝——判断是否异常跳变
    | measureReject.baroAlt_notJump = ...
    |     abs(norm(alt_pre-alt)) < posJumpThreshold;
    | % 气压高度位置跳变拒绝——判断是否异常跳变
    | measureReject.range_notJump = ...
    |     abs(norm(range_pre-range)) < posJumpThreshold;
    | %% 残差拒绝
    | % ublox1
    | [res_ublox1, resCov_ublox1] = residualgps(objMARG, mSensor_ublox1_lla, ...
    |     Rpos, mSensor_ublox1_gpsvel, Rvel);
    | normalizedRes_ublox1 = res_ublox1 ./ sqrt( diag(resCov_ublox1).' );
    | residual_ublox1 = any(abs(normalizedRes_ublox1(1:3))<6);
    | if ~residual_ublox1
    |     ublox1_resReject_num = ublox1_resReject_num + 1;
    | end
    | % um482
    | [res_um482, resCov_um482] = residualgps(objMARG, mSensor_um482_lla, ...
    |     Rpos_um482, mSensor_um482_gpsvel, Rvel_um482);
    | normalizedRes_um482 = res_um482 ./ sqrt( diag(resCov_um482).' );
    | switch mThis_bestpos
    |     case ENUM_BESTPOS.POS_SOLUTION_NARROW_INT % 高精度解
    |         residual_um482 = any(abs(normalizedRes_um482(1:3))<100);
    |     case ENUM_BESTPOS.POS_SOLUTION_SINGLE
    |         residual_um482 = any(abs(normalizedRes_um482(1:3))<10);
    |     case ENUM_BESTPOS.POS_SOLUTION_NONE
    |         residual_um482 = false;
    |     otherwise
    |         residual_um482 = any(abs(normalizedRes_um482(1:3))<100);
    | end
    | if ~residual_um482
    |     um482_resReject_num = um482_resReject_num + 1;
    | end
    | % mag
    | [res_mag, resCov_mag] = residualmag(objMARG, mag, Rmag);
    | normalizedRes_mag = res_mag./ sqrt( diag(resCov_mag).' );
    | residual_mag = all( abs(normalizedRes_mag)<10 );
    | if ~residual_mag
    |     deciMag = 12;
    | else
    |     deciMag = 3;
    |     mag_resReject_num = mag_resReject_num + 1;
    |     if mag_resReject_num > 1e6 % 如果拒绝次数过多，则认定传感器失效，永久拒绝
    |         %         magRejectForEver = true;
    |     end
    | end
    | %% 瞬时静止判定
    | StillCondition.acc = abs(accel(1)) < 0.5 && abs(accel(2)) < 0.5; % 横向加速度小于阈值
    | StillCondition.gyro = max(gyro)<0.05; % rad
    | StillCondition.gpsvel = (max(abs(mSensor_ublox1_gpsvel))<0.2 && ...
    |     mIntegrity_status_ublox1 == ENUM_SensorHealthStatus.Health) || ...
    |     (max(abs(mSensor_um482_gpsvel))<0.2 && ...
    |     mIntegrity_status_um482 == ENUM_SensorHealthStatus.Health); % m/s
    | StillCondition.isStatic = false;
    | StillCondition.isStatic = StillCondition.acc && ...
    |     StillCondition.gyro && ...
    |     StillCondition.gpsvel;
    | ZVCenable = false;
    | if StillCondition.isStatic && MARGParam.enableZeroVelCorrect
    |     staticTime = staticTime + Ts;
    |     if staticTime > 2
    |         ZVCenable = true; % 零速校正使能
    |     end
    | else
    |     staticTime = 0;
    | end
    | %% 滤波
    | disenable_time = clock_sec < 150 || clock_sec > inf;
    | disenable_time = true;
    | enable_gps_time = clock_sec < 3049;
    | enable_gps_time = true;
    | 
    | ublox1_is_available = ...
    |     mIntegrity_status_ublox1 == ENUM_SensorHealthStatus.Health || ...
    |     mIntegrity_status_ublox1 == ENUM_SensorHealthStatus.Degrade;
    | um482_is_available = ...
    |     mIntegrity_status_um482 == ENUM_SensorHealthStatus.Health || ...
    |     mIntegrity_status_um482 == ENUM_SensorHealthStatus.Degrade;
    | airspeed1_is_available = ...
    |     mIntegrity_status_airspeed1 == ENUM_SensorHealthStatus.Health;
    | mag_is_available = ...
    |     mIntegrity_status_mag1 == ENUM_SensorHealthStatus.Health || ...
    |     mIntegrity_status_mag2 == ENUM_SensorHealthStatus.Health;
    | baro_is_available = ...
    |     mIntegrity_status_baro1 == ENUM_SensorHealthStatus.Health;
    | isLatLonAvailable = ...
    |     ~(~ublox1_is_available && ~um482_is_available);
    | isHeightAvailable = ~(~baro_is_available && ~ublox1_is_available && ~um482_is_available);
    | %% IMU 过程更新
    | step_imu = step_imu + 1;
    | temp_gyro = 3;
    | temp_acc = 3;
    | meanAcc = (temp_acc-1)/temp_acc*meanAcc+1/temp_acc*accel;
    | meanGyro = (temp_gyro-1)/temp_gyro*meanGyro+1/temp_gyro*gyro;
    | if rem(step_imu,deciIMU) == 0
    |     % 在旋翼转固定翼模式进行加计方差放大（V1000在该模式中垂向加计会出现很大的测量偏差）
    |     objMARG.AccelerometerBiasNoise = MARGParam.std_acc_bias.^2;
    |     objMARG.AccelerometerNoise = MARGParam.std_acc.^2;
    |     if MARGParam.enableAccDegrade_Rotor2Fix
    |         if mTask_taskMode == ENUM_FlightTaskMode.Rotor2Fix_Mode
    |             objMARG.AccelerometerBiasNoise = 2e2*MARGParam.std_acc_bias.^2;
    |             objMARG.AccelerometerNoise = 5*MARGParam.std_acc.^2;
    |         else
    |             objMARG.AccelerometerBiasNoise = MARGParam.std_acc_bias.^2;
    |             objMARG.AccelerometerNoise = MARGParam.std_acc.^2;
    |             if preTaskMode == ENUM_FlightTaskMode.Rotor2Fix_Mode && mTask_taskMode ~= ENUM_FlightTaskMode.Rotor2Fix_Mode
    |                 fprintf('Rotor2Fix Complete!\n');
    |                 isRotor2FixComplete = true;
    |                 objMARG.State(14:16) = 0.1*objMARG.State(14:16); % 加计零偏重置
    |             end
    |         end
    |     end
    |     objMARG.GyroscopeBiasNoise = MARGParam.std_gyro_bias.^2;
    |     objMARG.GyroscopeNoise = MARGParam.std_gyro.^2;
    |     % 根据垂向加计的幅值进行加计方差的修正 (不好, 后续应废弃)
    |     tmpK_residual = [1,1,1];
    |     for ii = 3
    |         if ii == 3
    |             tmpK_bias = max(1,(abs(abs(meanAcc(ii))-9.8)/1)^1.5);
    |             tmpK = max(1,(abs(abs(meanAcc(ii))-9.8)/1)^3);
    |         else
    |             tmpK_bias = max(1,abs(meanAcc(ii))^1.5);
    |             tmpK = max(1,abs(meanAcc(ii))^3);
    |         end
    |         % fprintf('tmpK_bias: %f\ttmpK: %f\n',tmpK_bias,tmpK);
    |         objMARG.AccelerometerBiasNoise(ii) = tmpK_residual(ii)*tmpK_bias*objMARG.AccelerometerBiasNoise(ii);
    |         objMARG.AccelerometerNoise(ii) = tmpK_residual(ii)*tmpK*objMARG.AccelerometerNoise(ii);
    |     end
    |     for ii = 1:3
    |         tmpK = (1+1*abs(meanGyro(ii)))^2;
    |         objMARG.GyroscopeBiasNoise = tmpK*MARGParam.std_gyro_bias.^2;
    |         objMARG.GyroscopeNoise = tmpK*MARGParam.std_gyro.^2;
    |     end
    |     % 根据加计测量方差对加计滤波方差进行修正
    |     tempAcc = mSensor_IMU1_acc;
    |     tempAz = tempAcc(3);
    |     [~,kAz] = smoothstd(tempAz);
    |     kAz = kAz^2;
    |     if kAz < 1
    |         kAz = 1;
    |     end
    |     for ii = 1:3
    |         objMARG.AccelerometerBiasNoise(ii) = kAz*objMARG.AccelerometerBiasNoise(ii);
    |         objMARG.AccelerometerNoise(ii) = kAz/2*objMARG.AccelerometerNoise(ii);
    |     end
    |     % 过程更新
    |     fuseAcc = meanAcc;
    |     fuseGyro = meanGyro;
    |     objMARG.predict(fuseAcc,fuseGyro);  %
    | end
    | %% 磁力计测量更新
    | if disenable_time && mag_is_available && ~magRejectForEver && magUpdateFlag && MARGParam.fuse_enable.mag % mag 更新
    |     step_mag = step_mag + 1;
    |     if rem(step_mag,deciMag) == 0
    |         objMARG.fusemag(mag,Rmag);
    |     end
    |     %% 利用磁力计/加计计算粗姿态辅助更新姿态四元数，防止初始化过程造成的一些问题
    |     enableMagQuatFuse = false;
    |     if enableMagQuatFuse &&                                      ... % 使能
    |             StillCondition.isStatic &&                       ... % 静态
    |             mTask_taskMode == ENUM_FlightTaskMode.GroundStandByMode && ... % 地面模式
    |             rem(step_mag,10) == 0                                ... % 间隔执行
    |         quat_ecompass = compact(ecompass(meanAcc,mag));
    |         eulerd_ecompass = euler(quat_ecompass)*180/pi + magDec_deg;
    |         for i_q = 1:4
    |             Rq = 0.05^2;
    |             objMARG.correct(i_q,quat_ecompass(i_q),Rq);
    |         end
    |     end
    | end
    | if rem(step,10) == 0 && mag_is_available
    |     quat_ecompass = compact(ecompass(meanAcc,mag));
    |     pEulerd_ecompass = euler(quat_ecompass)*180/pi + magDec_deg;
    | end
    | %% ublox1 测量更新
    | if enable_gps_time && ublox1_is_available && measureReject.ublox1_lla_notJump && ...
    |         mIntegrity_update_ublox1 && MARGParam.fuse_enable.gps
    |     step_ublox = step_ublox + 1;
    |     if ~ZVCenable
    |         if rem(step_ublox,deciUblox) == 0
    |             objMARG.fusegps(mSensor_ublox1_lla,Rpos,mSensor_ublox1_gpsvel,Rvel);
    |         end
    |     else
    |         if rem(step_ublox,deciUblox) == 0
    |             objMARG.fusegps(mSensor_ublox1_lla,Rpos,[0,0,0],Rvel);
    |         end
    |     end
    | end
    | %% um482 测量更新
    | hasBigError = isRtkHasBigErrorWithUblox(mSensor_ublox1_ll,...
    |                           mSensor_um482_ll,...
    |                           mIntegrity_status_ublox1 == ENUM_SensorHealthStatus.Health);
    | if enable_gps_time && ... % 调试
    |         ~hasBigError && ... % ublox与rtk定位差异过大，可能由于rtk错误造成
    |         MARGParam.fuse_enable.um482 && ...
    |         um482_is_available && ...
    |         mIntegrity_update_um482 && ...% gps 更新
    |         mThis_bestpos ~= ENUM_BESTPOS.POS_SOLUTION_NONE && ...% 无解
    |         mSensor_um482_pdop ~= 0 % um482在受强干扰时pDop会置0
    |     objMARG.fusegps(mSensor_um482_lla,Rpos_um482,mSensor_um482_gpsvel,Rvel_um482);
    | end
    | %% 雷达高融合（未使用）
    | if false && radarUpdateFlag && measureReject.range_notJump  %
    |     step_radar = step_radar + 1;
    |     if rem(step_radar,deciRadar) == 0
    |         idx_alt = 7; % 高度的状态序号
    |         posd = -range-dHeight_GPS_sub_Baro;
    |         Rposd = Rrange;
    |         objMARG.correct(idx_alt,posd,Rposd);
    |     end
    | end
    | %% 气压高测量更新
    | isFuseBaroAlt = baroUpdateFlag && measureReject.baroAlt_notJump && MARGParam.fuse_enable.alt && ...% 当ublox失效且baro正常时执行
    |     MARGParam.fuse_enable.gps && ...
    |     ~isLatLonAvailable;
    | if isLatLonAvailable % gps恢复后，重置baro融合次数
    |     idxFuseBaro = 0;
    | end
    | if isFuseBaroAlt
    |     idxFuseBaro = idxFuseBaro + 1;
    |     if idxFuseBaro == 1 || idxFuseBaro == 2 % 融合的初始阶段，放大高度估计方差，防止垂速估计偏离
    |         objMARG.StateCovariance(7,7) = max(10^2,objMARG.StateCovariance(7,7));
    |     end
    |     step_baro = step_baro + 1;
    |     if rem(step_baro,deciBaro) == 0
    |         idx_alt = 7; % 高度的状态序号
    |         posd = -alt-dHeight_GPS_sub_Baro;
    |         Rposd = Ralt;
    |         objMARG.correct(idx_alt,posd,Rposd);
    |     end
    | end
    | %% 真空速测量更新（进行风估计）
    | if airspeedUpdateFlag && ...
    |         airspeed1_is_available
    |     step_tas = step_tas + 1;
    |     kTAS = 0.9;
    |     preTAS = kTAS*preTAS + (1-kTAS)*tas;
    |     if rem(step_tas,deciAirspeed) == 0
    |         if nState == 24
    |             objMARG.fuseTAS(preTAS,Rtas);
    |         else
    |             
    |         end                
    |     end
    | end
    | %% 空速测量更新
    | if airspeedUpdateFlag && ...
    |         airspeed1_is_available && ...
    |         ~isLatLonAvailable % || clock_sec >= 700% || clock_sec >= 700
    |     % 当GPS失效时，引入空速，抑制融合速度的漂移
    |     tempLLA = objMARG.ReferenceLocation;
    |     Rvel_airspeed = diag([7,7,25]).^2;
    |     stateEst = objMARG.State;
    |     euler_rad = euler(stateEst(1:4));
    |     yaw = euler_rad(1) + 5*randn/3/57.3;
    |     pitch = euler_rad(2);
    |     DCMbe = [cos(pitch) 0 -sin(pitch);0 1 0;sin(pitch) 0 cos(pitch)]*[cos(yaw) sin(yaw) 0;-sin(yaw) cos(yaw) 0;0 0 1]; % NED到Body的坐标转换矩阵
    |     DCMeb = DCMbe'; % Body到NED的坐标转换矩阵
    |     vel_airspeed = (DCMeb*[tas;0;0])';
    |     objMARG.fusegps(tempLLA,1e10,vel_airspeed,Rvel_airspeed);
    | end
    | %%
    | if nState == 24
    |     stateEst = [objMARG.State];
    | else
    |     stateEst = [objMARG.State;0;0];
    | end
    | 
    | if ~isFuseBaroAlt
    |     % 补偿平面坐标系造成的高度偏差
    |     distFromOri = norm(stateEst(5:6));
    |     R0 = 6378.137e3;
    |     H0 = norm([R0,distFromOri]);
    |     dH = H0 - R0;
    |     stateEst(7) = stateEst(7) - dH; % 高度处理
    | end
    | if nState == 24
    |     stateCovarianceDiagEst = [abs(diag(objMARG.StateCovariance)).^0.5];
    | else
    |     stateCovarianceDiagEst = [abs(diag(objMARG.StateCovariance)).^0.5;0;0];
    | end
    | eulerd = euler(stateEst(1:4))*180/pi;
    | posNED = stateEst(5:7)';
    | % lla_out = flat2lla_codegen(posNED, refloc(1:2), 0, refloc(3));
    | lla_out = flat2lla_codegen(posNED, NaviFilterOut.InitValue.refloc(1:2), 0, 0); % href: flat的高度基准，向下为正
    | if MARGParam.enableVdFuser && ...
    |         (mIntegrity_status_ublox1 == ENUM_SensorHealthStatus.Health && range > 8)
    |     k = max(1,abs(accel(3)-9.8));
    |     temp = min(0.2,1/k^0.8);
    |     if mIntegrity_status_ublox1 == ENUM_SensorHealthStatus.Health
    |         if mIntegrity_update_ublox1
    |             thisTime = clock_sec;
    |             dTime = thisTime - timeUpdate_ublox;
    |             timeUpdate_ublox = thisTime;
    |             kDTime = 0.9;
    |             pDTime = kDTime*pDTime + (1-kDTime)*dTime;
    |         end
    |         if pDTime < 0.25 % 更新率低时不进行平滑
    |             fuseVd = temp*stateEst(10) + (1-temp)*mSensor_ublox1_vd;
    |             stateEst(10) = fuseVd;
    |         end
    |     end
    | end
    | lla_pre = mSensor_ublox1_lla;
    | alt_pre = alt;
    | range_pre = range;
    | preTaskMode = mTask_taskMode;
    | step = step + 1;
    | %% 更新输出
    | NaviFilterOut.state = stateEst;
    | NaviFilterOut.stateCovariance = stateCovarianceDiagEst;
    | 
    | NaviFilterOut.quaternion = stateEst(1:4);
    | NaviFilterOut.posNED = stateEst(5:7);
    | NaviFilterOut.velNED = stateEst(8:10);
    | NaviFilterOut.dangle = stateEst(11:13);
    | NaviFilterOut.dvel = stateEst(14:16);
    | NaviFilterOut.magNED = stateEst(17:19);
    | NaviFilterOut.dmagB = stateEst(20:22);
    | NaviFilterOut.windNE = stateEst(23:24);
    | NaviFilterOut.dw = NaviFilterOut.dangle/Ts;
    | NaviFilterOut.dacc = NaviFilterOut.dvel/Ts;
    | NaviFilterOut.yawd = eulerd(1);
    | NaviFilterOut.pitchd = eulerd(2);
    | NaviFilterOut.rolld = eulerd(3);
    | NaviFilterOut.eulerd_yaw_pitch_roll = eulerd';
    | NaviFilterOut.latd = lla_out(1);
    | NaviFilterOut.lond = lla_out(2);
    | NaviFilterOut.alt = lla_out(3);
    | NaviFilterOut.lla = lla_out';
    | NaviFilterOut.eulerd_ecompass = pEulerd_ecompass;
    | NaviFilterOut.accel_correct = meanAcc' - NaviFilterOut.dacc;
    | NaviFilterOut.gyro_correct = meanGyro' - NaviFilterOut.dw;
    | 
    | NaviFilterOut.Covariance.P_quaternion = stateCovarianceDiagEst(1:4);
    | NaviFilterOut.Covariance.P_posNED = stateCovarianceDiagEst(5:7);
    | NaviFilterOut.Covariance.P_velNED = stateCovarianceDiagEst(8:10);
    | NaviFilterOut.Covariance.P_dangle = stateCovarianceDiagEst(11:13);
    | NaviFilterOut.Covariance.P_dvel = stateCovarianceDiagEst(14:16);
    | NaviFilterOut.Covariance.P_magNED = stateCovarianceDiagEst(17:19);
    | NaviFilterOut.Covariance.P_dmagB = stateCovarianceDiagEst(20:22);
    | NaviFilterOut.Covariance.P_windNE = stateCovarianceDiagEst(23:24);
    | NaviFilterOut.Status.nUbloxRejectByResidual = ublox1_resReject_num;
    | NaviFilterOut.Status.nUm482RejectByResidual = um482_resReject_num;
    | NaviFilterOut.Status.nMagRejectByResidual = mag_resReject_num;
    | NaviFilterOut.Status.isLatLonAvailable = isLatLonAvailable;
    | NaviFilterOut.Status.isHeightAvailable = isHeightAvailable;
    | NaviFilterOut.innovMARG.ublox1 = normalizedRes_ublox1;
    | NaviFilterOut.innovMARG.um482 = normalizedRes_um482;
    | NaviFilterOut.innovMARG.mag = normalizedRes_mag;
    | NaviFilterOut.innovMARG.baro = 0;
    | NaviFilterOut.innovMARG.radar = 0;
    | NaviFilterOut.stepInfo.step = step;
    | NaviFilterOut.stepInfo.step_imu = step_imu;
    | NaviFilterOut.stepInfo.step_mag = step_mag;
    | NaviFilterOut.stepInfo.step_ublox = step_ublox;
    | NaviFilterOut.stepInfo.step_radar = step_radar;
    | NaviFilterOut.stepInfo.step_baro = step_baro;
    | NaviFilterOut.stepInfo.step_board = step_board;
    | end
    | %% 子函数
    | function eout = euler(quat)
    | % rotate 'ZYX'
    | qa = quat(1);
    | qb = quat(2);
    | qc = quat(3);
    | qd = quat(4);
    | the1 = 1;
    | the2 = 2;
    | 
    | tmp = qb.*qd.*the2 - qa.*qc.*the2;
    | if tmp > the1
    |     tmp = the1;
    | elseif tmp < -the1
    |     tmp = -the1;
    | end
    | % tmp(tmp > the1) = the1;
    | % tmp(tmp < -the1) = -the1;
    | b = -asin(tmp);
    | a = atan2((qa.*qd.*the2 + qb.*qc.*the2),(qa.^2.*the2 - the1 + qb.^2.*the2));
    | c = atan2((qa.*qb.*the2 + qc.*qd.*the2),(qa.^2.*the2 - the1 + qd.^2.*the2));
    | eout = [a b c];
    | end
    | %%
    | function lla = flat2lla_codegen(p, ll0, psi0, href)
    | lla = zeros(1,3);
    | R = 6378.137e3;
    | f = 0.003352810664747;
    | %     % wrap latitude and longitude if needed
    | %     [~, ll0(1), ll0(2)] = wraplatitude( ll0(1), ll0(2), 'deg' );
    | %
    | %     % check and fix angle wrapping in longitude
    | %     [~, ll0(2)] = wraplongitude( ll0(2), 'deg', '180' );
    | 
    | rll0 = ll0*pi/180;
    | rpsi0 = psi0*pi/180;
    | 
    | dNorth = cos(rpsi0)*p(:,1) - sin(rpsi0)*p(:,2);
    | dEast  = sin(rpsi0)*p(:,1) + cos(rpsi0)*p(:,2);
    | lla(:,3) = -p(:,3) - href;
    | 
    | Rn = R/sqrt(1-(2*f-f*f)*sin(rll0(1))*sin(rll0(1)));
    | Rm = Rn*((1-(2*f-f*f))/(1-(2*f-f*f)*sin(rll0(1))*sin(rll0(1))));
    | 
    | dLat = dNorth.*atan2(1,Rm);
    | dLon = dEast.*atan2(1,Rn*cos(rll0(1)));
    | 
    | lla(:,1) = dLat*180/pi + ll0(1);
    | lla(:,2) = dLon*180/pi + ll0(2);
    | 
    | %     % wrap latitude and longitude if needed
    | %     [~, lla(:,1), lla(:,2)] = wraplatitude( lla(:,1)', lla(:,2)', 'deg' );
    | %
    | %     % check and fix angle wrapping in longitude
    | %     [~, lla(:,2)] = wraplongitude( lla(:,2), 'deg', '180' );
    | end
    | %%
    | function flag = isReInitMagState(thisMagNum,taskMode,clock_sec)
    | persistent preMagNum
    | if isempty(preMagNum)
    |     preMagNum = thisMagNum;
    | end
    | flag = false;
    | if isempty(preMagNum)
    |     preMagNum = thisMagNum;
    | end
    | if thisMagNum == preMagNum
    |     isTheSameMag = true;
    | else
    |     isTheSameMag = false;
    | end
    | if taskMode == ENUM_FlightTaskMode.GroundStandByMode && ...
    |         clock_sec < 50 && ~isTheSameMag
    |     flag = true; 
    |     fprintf('time %.3f [sec]: Navigation Filter ReInit\n',clock_sec);
    | end
    | 
    | preMagNum = thisMagNum;
    | end
    | %% 更新 ublox 的测量协方差矩阵 
    | function [Rpos, Rvel] = getUbloxR()
    | posVec = mSensor_ublox1_pacc;
    | velVec = mSensor_ublox1_sacc*ones(1,3);
    | for i = 1:3
    |     if posVec(i) < MARGParam.std_lla(i) % 限制位置测量精度最低值
    |         posVec(i) = MARGParam.std_lla(i);
    |     end
    |     if velVec(i) < MARGParam.std_gpsvel(i) % 限制速度测量精度最低值
    |         velVec(i) = MARGParam.std_gpsvel(i);
    |     end
    | end
    | Rpos = diag(posVec.^2);
    | Rvel = diag(velVec.^2);
    | end
    | %% 更新 um482 的测量协方差矩阵  
    | function [Rpos_um482, Rvel_um482] = getUm482R(Rpos_um482, Rvel_um482)
    | switch mThis_bestpos
    |     case ENUM_BESTPOS.POS_SOLUTION_NARROW_INT % 高精度解
    |         sigmaLat = max(0.3,mSensor_um482_pacc(1));
    |         sigmaLon = max(0.3,mSensor_um482_pacc(2));
    |         sigmaAlt = max(0.3,mSensor_um482_pacc(3));
    |     case ENUM_BESTPOS.POS_SOLUTION_NARROW_FLOATE
    |         sigmaLat = 1e1*max(0.8,mSensor_um482_pacc(1));
    |         sigmaLon = 1e1*max(0.8,mSensor_um482_pacc(2));
    |         sigmaAlt = 1e1*max(0.6,mSensor_um482_pacc(3));
    |     otherwise % 其他可用解
    |         sigmaLat = max(0.6,mSensor_um482_pacc(1));
    |         sigmaLon = max(0.6,mSensor_um482_pacc(2));
    |         sigmaAlt = max(0.6,mSensor_um482_pacc(3));
    | end
    | Rpos_um482 = diag([sigmaLat,sigmaLon,sigmaAlt]).^2;
    | if mSensor_um482_pdop > 1.4
    |     Rvel_um482 = mSensor_um482_pdop^1.5*Rvel_um482;
    | end
    | end
  function du_func_KalmanFilter(mode):
    | function du_func_KalmanFilter(mode)
    | % 组合导航滤波计算
    | switch mode
    | %     case 17
    | %         % MOV17
    | %         X0 = single([alignInitValue.quat0,[0,0,-alignInitValue.refloc(3)],alignInitValue.gpsvel0,alignInitValue.gyro_bias0,...
    | %             [0,0,0],1,zeros(1,5)]);
    | %         [NaviFilterOut.state,NaviFilterOut.stateCovariance,NaviFilterOut.eulerd,NaviFilterOut.lla,NaviFilterOut.innovMARG,NaviFilterOut.stepInfo] = ...
    | %             navi_mvo17(Ts,X0,alignInitValue.refloc,clock_sec,Sensors,SensorSignalIntegrity,ECASInfo,MVOParam,um482_BESTPOS,isBadAttitude);
    | %     case 24
    | %         % MARG24
    | %         [NaviFilterOut.state,NaviFilterOut.stateCovariance,NaviFilterOut.eulerd,NaviFilterOut.lla,NaviFilterOut.innovMARG,NaviFilterOut.stepInfo,ECASInfo] = ...
    | %             navi_marg24(Ts,X0,alignInitValue.refloc,clock_sec,Sensors,SensorSignalIntegrity,ECASInfo,MARGParam,um482_BESTPOS,isBadAttitude,mTask_taskMode);                    
    |     case 22
    |         % MARG22
    |         FilterMARG22();
    | otherwise
    |         % MARG22
    |         FilterMARG22();   
    | end
    | NaviFilterOut.Status.isHeadingRotateFlag = isHeadingRotate(NaviFilterOut.eulerd_yaw_pitch_roll(1)*pi/180,NaviFilterOut.eulerd_ecompass(1)*pi/180) ||...
    |     isMoving(NaviFilterOut.state(8:10));
    | NaviFilterOut.Status.isNavFilterGood = logical(NaviFilterOut.Status.initialAlignmentComplete);
  function flag = isRadarReady:
    | function flag = isRadarReady
    | persistent duration
    | if isempty(duration)
    |     duration = 0;
    | end
    | flag = true;
    | range = double(IN_Sensor.radar1.Range);
    | flag = range < 30 && IN_SignalIntegrity.SensorStatus.radar1 == ENUM_SensorHealthStatus.Health;
    | if ~flag
    |     duration = duration + Ts;
    |     if duration > 0.5
    |         isRadarReady = false; 
    |     end
    | end
  function [x_out,P_out,dz_out,Pz_out] = heightKalmanEst(Vd,height,Ts_in,reset,reject_threshold,Q,R,mode):
    | function [x_out,P_out,dz_out,Pz_out] = heightKalmanEst(Vd,height,Ts_in,reset,reject_threshold,Q,R,mode)
    | persistent x P dz Pz heightPre
    | if isempty(x) || reset
    |     x = height;
    |     P = 0.5;
    |     dz = 0;
    |     Pz = 0;
    |     heightPre = height;
    | end
    | u = -Vd;
    | z = height;
    | H = 1;
    | switch mode
    |     case 'predict'
    |         % 预测
    |         [x,P] = predict(x,u,Ts_in,P,Q);
    |     case 'fuse'
    |         % 矫正
    |         [x,P,dz,Pz] = fuseHeight(x,z,P,H,R,reject_threshold);
    | end
    | 
    | x_out = x;
    | P_out = P;
    | dz_out = dz;
    | Pz_out = Pz;
    | % 
    | heightPre = height;
    | %%
    | % 预测
    | function [x,P] = predict(x,u,Ts,P,Q)
    | x = x + u*Ts;
    | P = P + Q*Ts;
    | % 校正
    | function [x,P,dz,Pz] = fuseHeight(x,z,P,H,R,reject_threshold)
    | dz = z - x;
    | Pz = H*P*H'+R;
    | if abs(dz) < reject_threshold % 残差小于阈值
    |     K = P*H/(H*P*H'+R);
    |     P = (1-K*H)*P;
    |     P = (P+P')/2;    
    |     x = x + K*dz;
    | else
    |     % 残差超限拒绝测量值
    |     x = x;
    |     P = P;
    | end
    | % 测量信息更新
    | function flag = isHeightUpdate(height,heightPre)
    | if height ~= heightPre
    |     flag = true;
    | else
    |     flag = false;
    | end
  function du_func:
    | function du_func
    | % persistent height0ublox1 height0baro1 height0um482
    | % if isempty(height0ublox1)
    | %     height0ublox1 = 0;
    | %     height0baro1 = 0;
    | %     height0um482 = 0;
    | % end
    | persistent dz x P Pz
    | if isempty(dz)
    |     dz = 0;
    |     x = 0;
    |     P = 0;
    |     Pz = 0;
    | end
    | %%
    | ublox1_is_available = ...
    |     IN_SignalIntegrity.SensorStatus.ublox1 == ENUM_SensorHealthStatus.Health || ...
    |     IN_SignalIntegrity.SensorStatus.ublox1 == ENUM_SensorHealthStatus.Degrade;
    | um482_is_available = ...
    |     IN_SignalIntegrity.SensorStatus.um482 == ENUM_SensorHealthStatus.Health || ...
    |     IN_SignalIntegrity.SensorStatus.um482 == ENUM_SensorHealthStatus.Degrade;
    | baro1_is_available = IN_SignalIntegrity.SensorStatus.baro1 == ENUM_SensorHealthStatus.Health;
    | ublox1UpdateFlag = IN_SignalIntegrity.SensorUpdateFlag.ublox1;
    | heightUblox1 = double(IN_Sensor.ublox1.height);
    | um482UpdateFlag = IN_SignalIntegrity.SensorUpdateFlag.um482;
    | heightUm482 = double(IN_Sensor.um482.height);
    | baroUpdateFlag = IN_SignalIntegrity.SensorUpdateFlag.baro1;
    | heightBaro1 = double(IN_Sensor.baro1.alt_baro);
    | 
    | relHeightUblox1 = heightUblox1 - height0Ublox1;
    | relHeightUm482 = heightUm482 - height0Um482;
    | relHeightBaro1 = heightBaro1 - height0Baro1;
    | %%
    | radarUpdateFlag = IN_SignalIntegrity.SensorUpdateFlag.radar1;
    | heightRadar1 = double(IN_Sensor.radar1.Range);
    | reject_threshold = max(0.5,0.5*heightRadar1);
    | Vd_is_bad = false;
    | if ublox1_is_available
    |     Vd = double(IN_Sensor.ublox1.velD);
    | elseif um482_is_available
    |     Vd = double(IN_Sensor.um482.velD);
    | else
    |     Vd = 0;
    |     Vd_is_bad = true;
    | end
    | R = 0.2^2; % 高度测量偏差
    | if Vd_is_bad
    |     Q = 4;
    | else
    |     Q = 0.05^2; % Vd抖动偏差
    | end
    | [x,P,dz,Pz] = heightKalmanEst(Vd,heightRadar1,Ts,resetRadarFuser,reject_threshold,Q,R,'predict');
    | if radarUpdateFlag
    |     R = 0.05^2;
    |     [x,P,dz,Pz] = heightKalmanEst(Vd,heightRadar1,Ts,resetRadarFuser,reject_threshold,Q,R,'fuse');
    | end
    | if ublox1UpdateFlag && ublox1_is_available
    |     R = 0.2^2;
    |     [x,P,dz,Pz] = heightKalmanEst(double(IN_Sensor.ublox1.velD),relHeightUblox1,Ts,resetRadarFuser,10,Q,R,'fuse');
    | end
    | if um482UpdateFlag && um482_is_available
    |     R = 0.12^2;
    |     [x,P,dz,Pz] = heightKalmanEst(double(IN_Sensor.um482.velD),relHeightUm482,Ts,resetRadarFuser,10,Q,R,'fuse');
    | end    
    | % if radarUpdateFlag
    | %     [x,P,dz,Pz] = heightKalmanEst(Vd,relHeightBaro1,Ts,resetRadarFuser,reject_threshold,Vd_is_bad);
    | % end
    | %     
    | if abs(dz) > reject_threshold && ( ublox1_is_available || um482_is_available )
    |     % 异常情况，雷达高度与ublox的垂速出现较大不匹配
    |     x = x;
    | else
    |     % 正常情况，使用radar高降落
    | %     x = heightRadar1; 
    | end
    | resetRadarFuser = false;
    | RadarFilterOut.height = x;
    | RadarFilterOut.Pheight = P;
    | RadarFilterOut.dz = dz;
    | RadarFilterOut.Pz = Pz;
  function [mag,magUpdateFlag,isBagMag] = getScreeningMag:
    | function [mag,magUpdateFlag,isBagMag] = getScreeningMag
    | isBagMag = 0;
    | if mIntegrity_select_mag == 1
    |     magUpdateFlag = mIntegrity_update_mag1;
    |     mag = double(mSensor_mag1_mag);
    | elseif mIntegrity_select_mag == 2
    |     magUpdateFlag = mIntegrity_update_mag2;
    |     mag = double(mSensor_mag2_mag);
    | elseif mIntegrity_select_mag == 0
    |     magUpdateFlag = mIntegrity_update_mag1 & mIntegrity_update_mag2;
    |     mag = double(mSensor_mag1_mag+mSensor_mag2_mag)/2;
    | else % 随便预置一个地磁矢量
    |     magUpdateFlag = false;
    |     mag = [1,0,0];
    |     isBagMag = 1;
    | end
  function [tas,airspeedUpdateFlag] = getScreeningTAS:
    | function [tas,airspeedUpdateFlag] = getScreeningTAS()
    | if mIntegrity_select_airspeed == 1
    |     airspeedUpdateFlag = mIntegrity_update_airspeed1;
    |     tas = mSensor_airspeed1_ias;
    | elseif mIntegrity_select_airspeed == 2
    |     airspeedUpdateFlag = mIntegrity_update_airspeed2;
    |     tas = mSensor_airspeed2_ias;
    | elseif mIntegrity_select_airspeed == 3
    |     airspeedUpdateFlag = mIntegrity_update_airspeed3;
    |     tas = mSensor_airspeed3_ias;    
    | elseif mIntegrity_select_airspeed == 0
    |     airspeedUpdateFlag = mIntegrity_update_airspeed1 | mIntegrity_update_airspeed2;
    |     tas = (mSensor_airspeed1_ias+mSensor_airspeed2_ias)/2;
    | else % 
    |     airspeedUpdateFlag = false;
    |     tas = 0;
    | end
  function [alt,baroUpdateFlag] = getScreeningBaro:
    | function [alt,baroUpdateFlag] = getScreeningBaro
    | if mIntegrity_select_baro == 1
    |     baroUpdateFlag = mIntegrity_update_baro1;
    |     alt = mSensor_baro1_alt;
    | else % 
    |     baroUpdateFlag = mIntegrity_update_baro1;
    |     alt = mSensor_baro1_alt;
    | end
  function [range,radarUpdateFlag] = getScreeningRadar:
    | function [range,radarUpdateFlag] = getScreeningRadar
    | if mIntegrity_select_radar == 1
    |     radarUpdateFlag = mIntegrity_update_radar1;
    |     range = mSensor_radar1_range;
    | else % 
    |     radarUpdateFlag = mIntegrity_update_radar1;
    |     range = mSensor_radar1_range;
    | end
  function out = enumBESTPOS:
    | function out = enumBESTPOS()
    | val = mSensor_um482_bestpos;
    | switch val
    |     case 0
    |         out = ENUM_BESTPOS.POS_SOLUTION_NONE;
    |     case 16
    |         out = ENUM_BESTPOS.POS_SOLUTION_SINGLE;
    |     case 17
    |         out = ENUM_BESTPOS.POS_SOLUTION_PSRDIFF;
    |     case 48
    |         out = ENUM_BESTPOS.POS_SOLUTION_L1_INT;
    |     case 49
    |         out = ENUM_BESTPOS.POS_SOLUTION_WIDE_INT;
    |     case 50
    |         out = ENUM_BESTPOS.POS_SOLUTION_NARROW_INT;
    |     case 32
    |         out = ENUM_BESTPOS.POS_SOLUTION_L1_FLOATE;        
    |     case 34
    |         out = ENUM_BESTPOS.POS_SOLUTION_NARROW_FLOATE; 
    |     otherwise
    |         out = ENUM_BESTPOS.POS_SOLUTION_NONE;
    | end
